simulink model "model2_diagonal"  (R2024a)
settings: Solver=VariableStepAuto  StartTime=0.0  StopTime=10.0  RelTol=1e-3
settings Model: Creator=Professional  LastModifiedBy=Professional

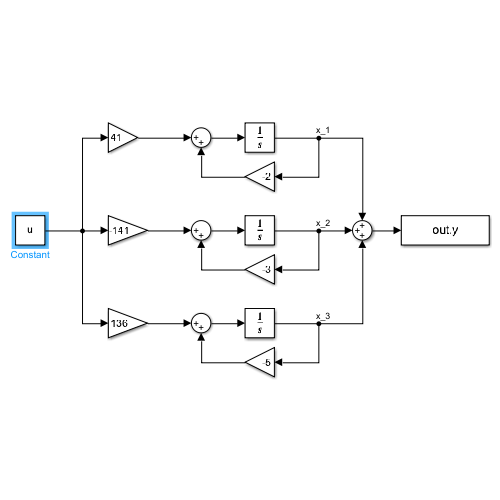
[thumbnail: Simulink's stored preview of the top-level diagram]
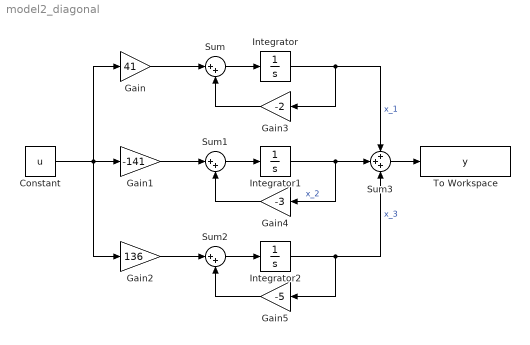
== system model2_diagonal ==
  Constant : Constant  Value=u  SampleTime=0.0001
  Gain : Gain  Gain=41
  Gain1 : Gain  Gain=-141
  Gain2 : Gain  Gain=136
  Gain3 : Gain  Gain=-2
  Gain4 : Gain  Gain=-3
  Gain5 : Gain  Gain=-5
  Integrator : Integrator
  Integrator1 : Integrator
  Integrator2 : Integrator
  Sum : Sum  Inputs=|++
  Sum1 : Sum  Inputs=|++
  Sum2 : Sum  Inputs=|++
  Sum3 : Sum  Inputs=+++
  To Workspace : ToWorkspace  VariableName=y  SaveFormat=Timeseries  SampleTime=-1
  wires:
  Constant/1 -> Gain2/1, Gain/1, Gain1/1
  Gain1/1 -> Sum1/1
  Gain/1 -> Sum/1
  Gain2/1 -> Sum2/1
  Sum/1 -> Integrator/1
  Sum1/1 -> Integrator1/1
  Sum2/1 -> Integrator2/1
  Integrator1/1 -> Gain4/1, Sum3/2  "x_2"
  Integrator/1 -> Sum3/1, Gain3/1  "x_1"
  Integrator2/1 -> Sum3/3, Gain5/1  "x_3"
  Gain3/1 -> Sum/2
  Gain5/1 -> Sum2/2
  Gain4/1 -> Sum1/2
  Sum3/1 -> To Workspace/1
